simulink model "Matrice_inertie_Mx"  (R2022b)
settings: Solver=VariableStepAuto  StartTime=0.0  StopTime=10.0  RelTol=1e-3
undefined symbols (not defined in the file): l1, l2, m1, m2
settings Model: Creator=cheye  LastModifiedBy=cheye

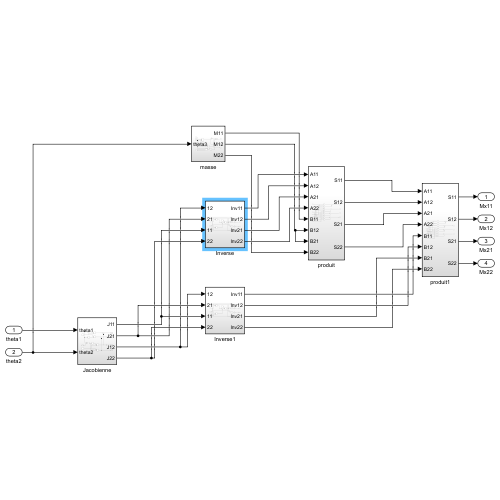
[thumbnail: Simulink's stored preview of the top-level diagram]
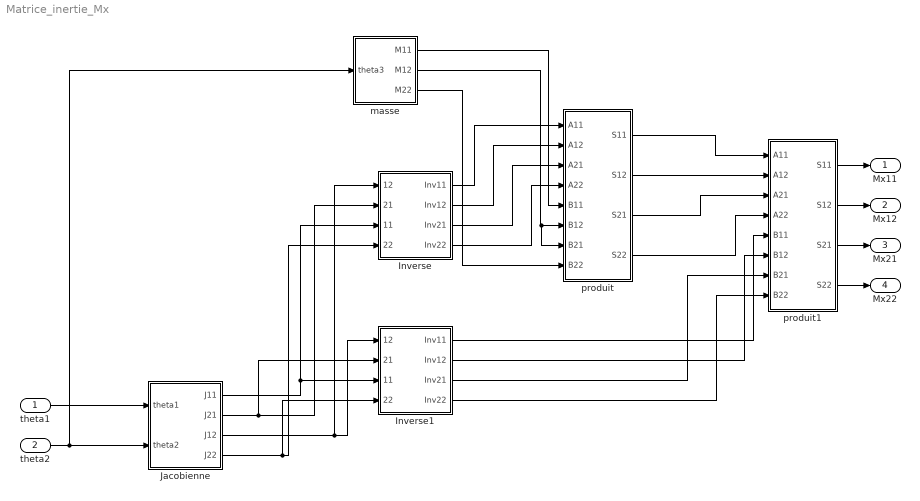
== system Matrice_inertie_Mx ==
  theta1 : Inport
  theta2 : Inport  Port=2
  Inverse : Subsystem
  Inverse1 : Subsystem
  Jacobienne : Subsystem
  masse : Subsystem
  produit : Subsystem
  produit1 : Subsystem
  Mx11 : Outport
  Mx12 : Outport  Port=2
  Mx21 : Outport  Port=3
  Mx22 : Outport  Port=4
  wires:
  theta1/1 -> Jacobienne/1(theta1)
  theta2/1 -> masse/1(theta3), Jacobienne/2(theta2)
  Jacobienne/1(J11) -> Inverse/3(11), Inverse1/3(11)
  Jacobienne/2(J21) -> Inverse1/2(21), Inverse/2(21)
  Jacobienne/3(J12) -> Inverse1/1(12), Inverse/1(12)
  Jacobienne/4(J22) -> Inverse1/4(22), Inverse/4(22)
  Inverse/1(Inv11) -> produit/1(A11)
  Inverse/2(Inv12) -> produit/2(A12)
  Inverse/3(Inv21) -> produit/3(A21)
  Inverse/4(Inv22) -> produit/4(A22)
  produit/1(S11) -> produit1/1(A11)
  produit/2(S12) -> produit1/2(A12)
  produit/3(S21) -> produit1/3(A21)
  produit/4(S22) -> produit1/4(A22)
  masse/1(M11) -> produit/5(B11)
  masse/2(M12) -> produit/7(B21), produit/6(B12)
  masse/3(M22) -> produit/8(B22)
  Inverse1/1(Inv11) -> produit1/5(B11)
  Inverse1/2(Inv12) -> produit1/6(B12)
  Inverse1/3(Inv21) -> produit1/7(B21)
  Inverse1/4(Inv22) -> produit1/8(B22)
  produit1/1(S11) -> Mx11/1
  produit1/2(S12) -> Mx12/1
  produit1/3(S21) -> Mx21/1
  produit1/4(S22) -> Mx22/1

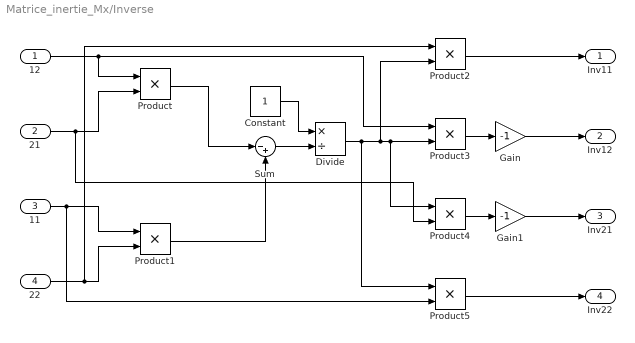
== system Matrice_inertie_Mx/Inverse ==
  12 : Inport
  21 : Inport  Port=2
  11 : Inport  Port=3
  22 : Inport  Port=4
  Constant : Constant
  Divide : Product  Inputs=*/
  Gain : Gain  Gain=-1
  Gain1 : Gain  Gain=-1
  Product{,1..5} (6 alike) : Product
  Sum : Sum  Inputs=|-+
  Inv11 : Outport
  Inv12 : Outport  Port=2
  Inv21 : Outport  Port=3
  Inv22 : Outport  Port=4
  wires:
  21/1 -> Product4/2, Product/2
  Product/1 -> Sum/1
  Divide/1 -> Product5/1, Product2/2, Product3/2, Product4/1
  22/1 -> Product1/2, Product2/1
  12/1 -> Product3/1, Product/1
  Product1/1 -> Sum/2
  11/1 -> Product5/2, Product1/1
  Constant/1 -> Divide/1
  Gain1/1 -> Inv21/1
  Product4/1 -> Gain1/1
  Product3/1 -> Gain/1
  Product5/1 -> Inv22/1
  Product2/1 -> Inv11/1
  Gain/1 -> Inv12/1
  Sum/1 -> Divide/2

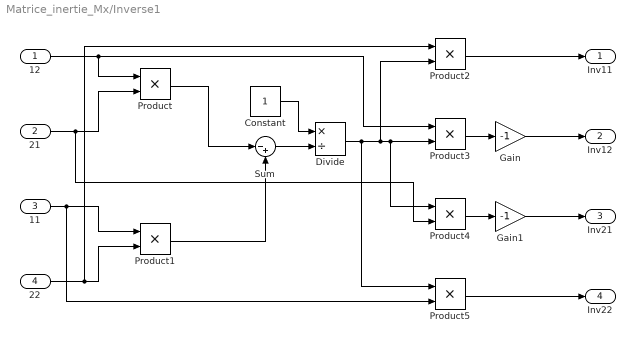
== system Matrice_inertie_Mx/Inverse1 ==
  12 : Inport
  21 : Inport  Port=2
  11 : Inport  Port=3
  22 : Inport  Port=4
  Constant : Constant
  Divide : Product  Inputs=*/
  Gain : Gain  Gain=-1
  Gain1 : Gain  Gain=-1
  Product{,1..5} (6 alike) : Product
  Sum : Sum  Inputs=|-+
  Inv11 : Outport
  Inv12 : Outport  Port=2
  Inv21 : Outport  Port=3
  Inv22 : Outport  Port=4
  wires:
  21/1 -> Product4/2, Product/2
  Product/1 -> Sum/1
  Divide/1 -> Product5/1, Product2/2, Product3/2, Product4/1
  22/1 -> Product1/2, Product2/1
  12/1 -> Product3/1, Product/1
  Product1/1 -> Sum/2
  11/1 -> Product5/2, Product1/1
  Constant/1 -> Divide/1
  Gain1/1 -> Inv21/1
  Product4/1 -> Gain1/1
  Product3/1 -> Gain/1
  Product5/1 -> Inv22/1
  Product2/1 -> Inv11/1
  Gain/1 -> Inv12/1
  Sum/1 -> Divide/2

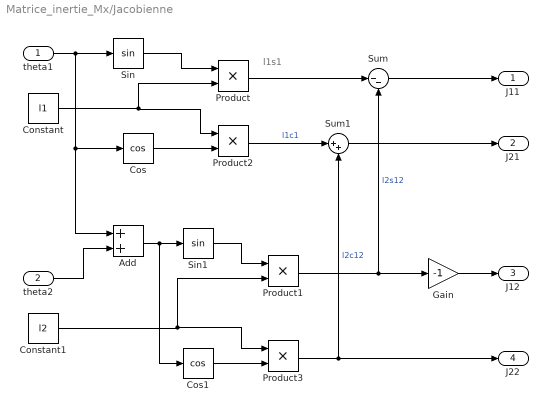
== system Matrice_inertie_Mx/Jacobienne ==
  note: l1s1
  theta1 : Inport
  theta2 : Inport  Port=2
  Add : Sum
  Constant : Constant  Value=l1
  Constant1 : Constant  Value=l2
  Cos : Trigonometry  Operator=cos
  Cos1 : Trigonometry  Operator=cos
  Gain : Gain  Gain=-1
  Product{,1..3} (4 alike) : Product
  Sin : Trigonometry
  Sin1 : Trigonometry
  Sum : Sum  Inputs=|--
  Sum1 : Sum  Inputs=|++
  J11 : Outport
  J21 : Outport  Port=2
  J12 : Outport  Port=3
  J22 : Outport  Port=4
  wires:
  Product3/1 -> J22/1, Sum1/2  "l2c12"
  Gain/1 -> J12/1
  Product1/1 -> Sum/2, Gain/1  "l2s12"
  Cos/1 -> Product2/2
  Add/1 -> Cos1/1, Sin1/1
  Constant/1 -> Product/2, Product2/1
  Sin/1 -> Product/1
  Constant1/1 -> Product3/1, Product1/2
  Cos1/1 -> Product3/2
  Sum1/1 -> J21/1
  theta1/1 -> Cos/1, Add/1, Sin/1
  theta2/1 -> Add/2
  Sin1/1 -> Product1/1
  Product2/1 -> Sum1/1  "l1c1"
  Product/1 -> Sum/1
  Sum/1 -> J11/1

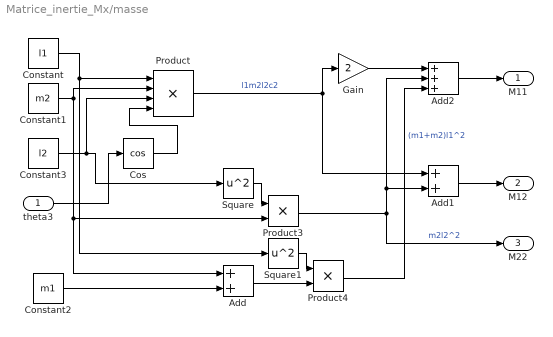
== system Matrice_inertie_Mx/masse ==
  theta3 : Inport
  Add : Sum
  Add1 : Sum
  Add2 : Sum  Inputs=+++
  Constant : Constant  Value=l1
  Constant1 : Constant  Value=m2
  Constant2 : Constant  Value=m1
  Constant3 : Constant  Value=l2
  Cos : Trigonometry  Operator=cos
  Gain : Gain  Gain=2
  Product : Product  Inputs=4
  Product3 : Product
  Product4 : Product
  Square : Math  Operator=square
  Square1 : Math  Operator=square
  M11 : Outport
  M12 : Outport  Port=2
  M22 : Outport  Port=3
  wires:
  Constant/1 -> Product/1, Square1/1
  Add2/1 -> M11/1
  Product/1 -> Add1/1, Gain/1  "l1m2l2c2"
  Constant1/1 -> Product/2, Add/1, Product3/2
  Constant3/1 -> Product/3, Square/1
  Cos/1 -> Product/4
  Product3/1 -> M22/1, Add2/2, Add1/2  "m2l2^2"
  Add/1 -> Product4/2
  Product4/1 -> Add2/3  "(m1+m2)l1^2"
  Constant2/1 -> Add/2
  Gain/1 -> Add2/1
  Square1/1 -> Product4/1
  Square/1 -> Product3/1
  theta3/1 -> Cos/1
  Add1/1 -> M12/1

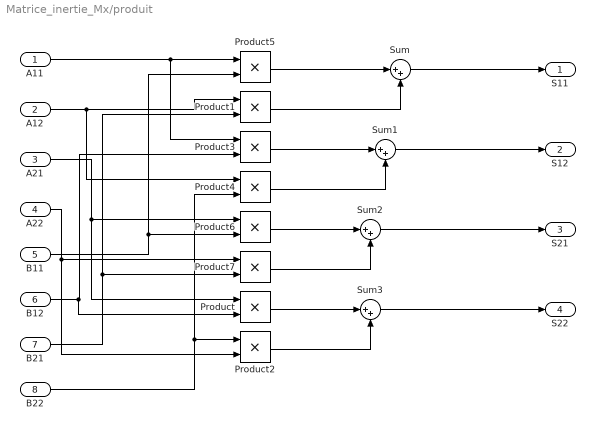
== system Matrice_inertie_Mx/produit ==
  A11 : Inport
  A12 : Inport  Port=2
  A21 : Inport  Port=3
  A22 : Inport  Port=4
  B11 : Inport  Port=5
  B12 : Inport  Port=6
  B21 : Inport  Port=7
  B22 : Inport  Port=8
  Product{,1..7} (8 alike) : Product
  Sum{,1..3} (4 alike) : Sum  Inputs=|++
  S11 : Outport
  S12 : Outport  Port=2
  S21 : Outport  Port=3
  S22 : Outport  Port=4
  wires:
  B21/1 -> Product7/2, Product1/2
  Product1/1 -> Sum/2
  B12/1 -> Product/2, Product3/2
  Product/1 -> Sum3/1
  B11/1 -> Product6/2, Product5/2
  Product2/1 -> Sum3/2
  A22/1 -> Product2/2, Product7/1
  A11/1 -> Product3/1, Product5/1
  Product7/1 -> Sum2/2
  A21/1 -> Product/1, Product6/1
  B22/1 -> Product2/1, Product4/2
  Product3/1 -> Sum1/1
  Product5/1 -> Sum/1
  A12/1 -> Product4/1, Product1/1
  Sum3/1 -> S22/1
  Sum/1 -> S11/1
  Product6/1 -> Sum2/1
  Product4/1 -> Sum1/2
  Sum2/1 -> S21/1
  Sum1/1 -> S12/1

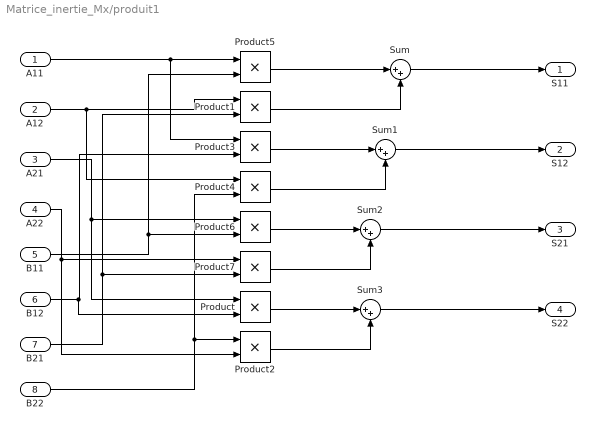
== system Matrice_inertie_Mx/produit1 ==
  A11 : Inport
  A12 : Inport  Port=2
  A21 : Inport  Port=3
  A22 : Inport  Port=4
  B11 : Inport  Port=5
  B12 : Inport  Port=6
  B21 : Inport  Port=7
  B22 : Inport  Port=8
  Product{,1..7} (8 alike) : Product
  Sum{,1..3} (4 alike) : Sum  Inputs=|++
  S11 : Outport
  S12 : Outport  Port=2
  S21 : Outport  Port=3
  S22 : Outport  Port=4
  wires:
  B21/1 -> Product7/2, Product1/2
  Product1/1 -> Sum/2
  B12/1 -> Product/2, Product3/2
  Product/1 -> Sum3/1
  B11/1 -> Product6/2, Product5/2
  Product2/1 -> Sum3/2
  A22/1 -> Product2/2, Product7/1
  A11/1 -> Product3/1, Product5/1
  Product7/1 -> Sum2/2
  A21/1 -> Product/1, Product6/1
  B22/1 -> Product2/1, Product4/2
  Product3/1 -> Sum1/1
  Product5/1 -> Sum/1
  A12/1 -> Product4/1, Product1/1
  Sum3/1 -> S22/1
  Sum/1 -> S11/1
  Product6/1 -> Sum2/1
  Product4/1 -> Sum1/2
  Sum2/1 -> S21/1
  Sum1/1 -> S12/1
